simulink model "vipfocus"  (R2015b)
settings: Solver=FixedStepDiscrete  StartTime=0.0  StopTime=inf  RelTol=1e-3
undefined symbols (not defined in the file or in its folder): gray, hot, magnitude
libraries: visiontextngfix x2, visionsinks x2, visiontransforms x1, vipmisc x1, dspvision x1
settings Model: FPTRunName=Active  Creator=The MathWorks, Inc.  LastModifiedBy=The MathWorks, Inc.
settings DataIOCC: LimitDataPoints=off  SaveFormat=Array  SaveOutput=off  SaveTime=off  SignalLoggingName=sigsOut
settings OptimizationCC: DefaultParameterBehavior=Inlined  InlineInvariantSignals=on  ExpressionDepthLimit=2147483647  InitFltsAndDblsToZero=on
settings DebuggingCC: SaveWithParameterizedLinksMsg=none  UnderspecifiedInitializationDetection=Classic  MergeDetectMultiDrivingBlocksExec=none  CheckExecutionContextPreStartOutputMsg=on  CheckExecutionContextRuntimeOutputMsg=on  SignalResolutionControl=TryResolveAllWithWarning  MultiTaskDSMMsg=warning  MultiTaskCondExecSysMsg=none  ParameterPrecisionLossMsg=none  FcnCallInpInsideContextMsg=UseLocalSettings  StateNameClashWarn=warning
settings HardwareCC: ProdBitPerPointer=32  ProdLargestAtomicFloat=None  ProdIntDivRoundTo=Undefined  ProdEndianess=Unspecified  ProdWordSize=32  ProdHWDeviceType=32-bit Generic  TargetBitPerLong=64  TargetBitPerPointer=64  TargetLongLongMode=on  TargetIntDivRoundTo=Zero  TargetEndianess=LittleEndian  TargetWordSize=64  TargetHWDeviceType=Generic->MATLAB Host Computer  ProdEqTarget=off
settings GRTTargetCC: TargetFcnLib=ansi_tfl_tmw.mat  GeneratePreprocessorConditionals=Disable all  CombineOutputUpdateFcns=off  GRTInterface=on
settings ConfigComp: CovModelRefEnable=Off

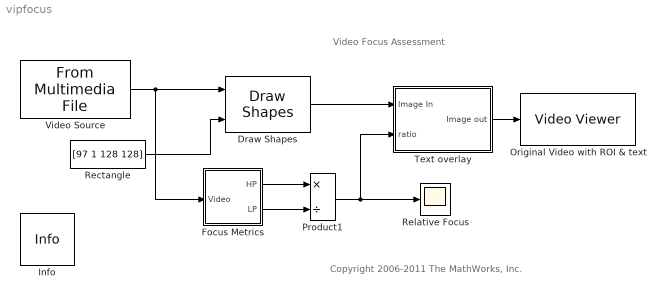
== system vipfocus ==
  note: Video Focus Assessment
  note: Copyright 2006-2011 The MathWorks, Inc.
  Draw Shapes : visiontextngfix/Draw Shapes  shape=Rectangles  fill=off  lineWidth=1  fillClrSource=Specify via dialog  display=Black  intensity=200  color=200  opacity=0.6  viewport=Entire image  antialiasing=off  inType=Obsolete  imagePorts=One multidimensional signal  prodOutputMode=Binary point scaling  prodOutputWordLength=32  prodOutputFracLength=14  memoryMode=Specify word length  memoryWordLength=16  memoryFracLength=15  roundingMode=Floor  overflowMode=off
  Focus Metrics : Subsystem
  Info : vipmisc/Info  SystemSampleTime=-1
  Original Video with ROI & text : visionsinks/Video Viewer  inputType=Obsolete7b  imagePorts=One multidimensional signal  useColorMap=off  colormapValue=gray(256)  specRange=off  minInputVal=0  maxInputVal=255  FigPos=[43 721 320 265]  AxisZoom=on  trueSizedOnce=on  OpenAtMdlStart=on  DefaultConfigurationName=vipscopes.VideoViewerScopeCfg
  Product1 : Product  Inputs=*/  SaturateOnIntegerOverflow=on  InputSameDT=on  OutDataTypeStr=Inherit: Same as first input
  Rectangle : Constant  Value=[97 1 128 128]  VectorParams1D=off
  Relative Focus : Scope
  Text overlay : Subsystem
  Video Source : dspvision/From Multimedia File  inputFilename=vipfly.avi  loop=on  numPlays=inf  outputStreams=Video and audio  videoDataType=single  audioDataType=int16  inheritSampleTime=on  userDefinedSampleTime=1/30  noAudioOutput=off  isIntensityVideo=off  fourcc=Intensity  colorVideoFormat=Separate color signals  outputEOF=off  dataOrg=Column-major  audioFrameSize=1024  computeAudioFrameSize=off  outSamplingMode=Frame based
  wires:
  Video Source/1 -> Focus Metrics/1(Video), Draw Shapes/1
  Focus Metrics/1(HP) -> Product1/1
  Focus Metrics/2(LP) -> Product1/2
  Product1/1 -> Text overlay/2(ratio), Relative Focus/1
  Text overlay/1(Image out) -> Original Video with ROI & text/1
  Draw Shapes/1 -> Text overlay/1(Image In)
  Rectangle/1 -> Draw Shapes/2

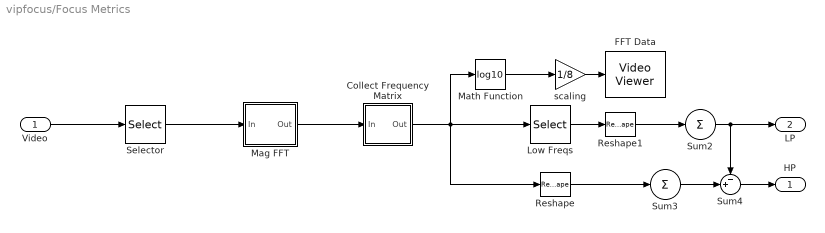
== system vipfocus/Focus Metrics ==
  Video : Inport
  Collect Frequency Matrix : Subsystem
  FFT Data : visionsinks/Video Viewer  inputType=Obsolete7b  imagePorts=One multidimensional signal  useColorMap=on  colormapValue=hot(256)  specRange=off  minInputVal=0  maxInputVal=8  FigPos=[728 324 121 121]  AxisZoom=on  trueSizedOnce=on  OpenAtMdlStart=on  DefaultConfigurationName=vipscopes.VideoViewerScopeCfg
  Low Freqs : Selector  NumberOfDimensions=2  InputPortWidth=3  IndexOptions=Index vector (dialog),Index vector (dialog)  Indices=[1:5],[1:5]  OutputSizes=1,1
  Mag FFT : Subsystem
  Math Function : Math  Operator=log10  SaturateOnIntegerOverflow=on
  Reshape : Reshape  OutputDimensionality=Column vector (2-D)
  Reshape1 : Reshape  OutputDimensionality=Column vector (2-D)
  Selector : Selector  NumberOfDimensions=2  InputPortWidth=3  IndexOptions=Index vector (dialog),Index vector (dialog)  Indices=[1:128],[97:(97+128-1)]  OutputSizes=1,1
  Sum2 : Sum  Inputs=1  SaturateOnIntegerOverflow=on  InputSameDT=on  OutDataTypeStr=Inherit: Same as first input
  Sum3 : Sum  Inputs=1  SaturateOnIntegerOverflow=on  InputSameDT=on  OutDataTypeStr=Inherit: Same as first input
  Sum4 : Sum  Inputs=-+|  SaturateOnIntegerOverflow=on  InputSameDT=on  OutDataTypeStr=Inherit: Same as first input
  scaling : Gain  Gain=1/8  SaturateOnIntegerOverflow=on  OutDataTypeStr=Inherit: Same as input  ParamDataTypeStr=Inherit: Same as input
  HP : Outport
  LP : Outport  Port=2
  wires:
  Reshape1/1 -> Sum2/1
  Math Function/1 -> scaling/1
  Sum4/1 -> HP/1
  Sum3/1 -> Sum4/2
  Sum2/1 -> LP/1, Sum4/1
  Reshape/1 -> Sum3/1
  Low Freqs/1 -> Reshape1/1
  Selector/1 -> Mag FFT/1(In)
  Video/1 -> Selector/1
  Collect Frequency Matrix/1(Out) -> Math Function/1, Low Freqs/1, Reshape/1
  Mag FFT/1(Out) -> Collect Frequency Matrix/1(In)
  scaling/1 -> FFT Data/1

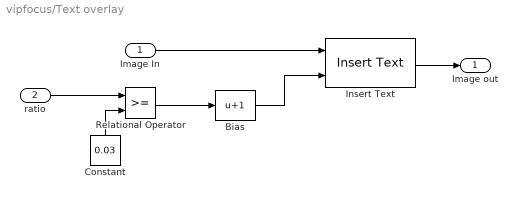
== system vipfocus/Text overlay ==
  Image In : Inport
  ratio : Inport  Port=2
  Bias : Bias  Bias=1
  Constant : Constant  Value=0.03  OutDataTypeStr=Inherit: Inherit via back propagation
  Insert Text : visiontextngfix/Insert Text  inputType=Obsolete  theText={'Out of focus','In focus'}  getTextLocFrom=Specify via dialog  textLoc="[100  10]"  getTextColorFrom=Specify via dialog  textColor=0  getTextIntensityFrom=Specify via dialog  textIntensity=0  getTextOpacityFrom=Specify via dialog  textOpacity=1.0  dummyVar2=0  dummyVar3=0  dummyVar4=0  imagePorts=One multidimensional signal  isInputTransposed=off  fontFace=LucidaSansRegular  dummyVar1=0  blockFontSize=16  antiAliased=on
  Relational Operator : RelationalOperator  OutDataTypeStr=fixdt(1,32)
  Image out : Outport
  wires:
  ratio/1 -> Relational Operator/1
  Constant/1 -> Relational Operator/2
  Insert Text/1 -> Image out/1
  Image In/1 -> Insert Text/1
  Relational Operator/1 -> Bias/1
  Bias/1 -> Insert Text/2

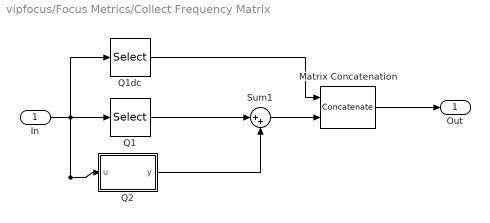
== system vipfocus/Focus Metrics/Collect Frequency Matrix ==
  In : Inport
  Matrix Concatenation : Concatenate  Mode=Multidimensional array  ConcatenateDimension=2
  Q1 : Selector  NumberOfDimensions=2  InputPortWidth=3  IndexOptions=Index vector (dialog),Index vector (dialog)  Indices=[1:16],[2:16]  OutputSizes=1,1
  Q1dc : Selector  NumberOfDimensions=2  InputPortWidth=3  IndexOptions=Index vector (dialog),Index vector (dialog)  Indices=[1:16],1  OutputSizes=1,1
  Q2 : MATLAB Function  TreatAsAtomicUnit=on
  Sum1 : Sum  Inputs=|++  SaturateOnIntegerOverflow=on  InputSameDT=on  OutDataTypeStr=Inherit: Same as first input
  Out : Outport
  wires:
  Q1/1 -> Sum1/1
  In/1 -> Q1dc/1, Q2/1(u), Q1/1
  Q1dc/1 -> Matrix Concatenation/1
  Sum1/1 -> Matrix Concatenation/2
  Matrix Concatenation/1 -> Out/1
  Q2/1(y) -> Sum1/2

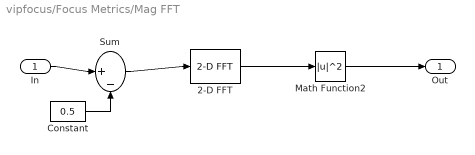
== system vipfocus/Focus Metrics/Mag FFT ==
  In : Inport
  2-D FFT : visiontransforms/2-D FFT  TableOpt=HYBRID  TableOptActive=Speed  BitRevOrder=off  SkipNorm=off  FFTImplementation=Auto  firstCoeffDataTypeStr=Inherit: Same word length as input  firstCoeffLastDataTypeStr=Inherit: Same word length as input  outputMin=[]  outputMax=[]  roundingMode=Floor  overflowMode=off
  Constant : Constant  Value=0.5  VectorParams1D=off  OutDataTypeStr=Inherit: Inherit via back propagation
  Math Function2 : Math  Operator=magnitude^2  SaturateOnIntegerOverflow=on
  Sum : Sum  Inputs=|+-  SaturateOnIntegerOverflow=on  InputSameDT=on  OutDataTypeStr=Inherit: Same as first input
  Out : Outport
  wires:
  Constant/1 -> Sum/2
  Sum/1 -> 2-D FFT/1
  2-D FFT/1 -> Math Function2/1
  In/1 -> Sum/1
  Math Function2/1 -> Out/1

== matlab function vipfocus/Focus Metrics/Collect Frequency Matrix/Q2 ==
  data: u input; y output
function y = fcn(u)
%#codegen

s = size(u);
colBegin = s(2)-14;
y = fliplr(u(1:16,colBegin:s(2)));
